simulink model "rmturretmodelrelease"  (R2025b)
settings: Solver=FixedStepAuto  StartTime=0.0  StopTime=tf  FixedStep=minstep  MaxStep=maxstep  MinStep=minstep  RelTol=tol  AbsTol=tol
values from neighbouring files (symbols this model uses):
  adecel = .4 * voltmax * kt * gearrat/(J * ra)    (= 19.7149704598)    [rmturretrelease.m]
  ascale = .9    (= 0.9)    [rmturretrelease.m]
  c = 5.526    [rmturretrelease.m]
  damp = .4    (= 0.4)    [rmturretrelease.m]
  dfreq = 3.7    [rmturretrelease.m]
  gearrat = 1    [rmturretrelease.m]
  intthresh = voltmax*.65    (= 15.6)    [rmturretrelease.m]
  ivmax = .8 / kiv    (= 0.016)    [rmturretrelease.m]
  J = 0.04145    [rmturretrelease.m]
  ka = J/(kt*gearrat)    (= 0.0559379217274)    [rmturretrelease.m]
  kb = .763 * g2    (= 0.763)    [rmturretrelease.m]
  kiv = 50    [rmturretrelease.m]
  kp = 23    [rmturretrelease.m]
  kpv = .01    (= 0.01)    [rmturretrelease.m]
  ks = uk /(kt*gearrat)    (= 1)    [rmturretrelease.m]
  kt = .741 * g2    (= 0.741)    [rmturretrelease.m]
  kv = kb*gearrat    (= 0.763)    [rmturretrelease.m]
  kvis = c/(kt*gearrat)    (= 7.45748987854)    [rmturretrelease.m]
  la = .00578 * 2    (= 0.01156)    [rmturretrelease.m]
  lat = .004    (= 0.004)    [rmturretrelease.m]
  namp = 0.0000000001    (= 1e-10)    [rmturretrelease.m]
  ra = 8.705    [rmturretrelease.m]
  squiggle = 0    [rmturretrelease.m]
  squigglefreq = 3    [rmturretrelease.m]
  testvel = 0    [rmturretrelease.m]
  theta0 = deg2rad(0)    [rmturretrelease.m]
  thetadotbreak = 6    [rmturretrelease.m]
  thetadotic = 0    [rmturretrelease.m]
  thetadotinput = 0    [rmturretrelease.m]
  thetatarget = deg2rad(170)    [rmturretrelease.m]
  Tpc = 1/500    (= 0.002)    [rmturretrelease.m]
  uk = .741    (= 0.741)    [rmturretrelease.m]
  vdt = 0    [rmturretrelease.m]
  veltar = 10    [rmturretrelease.m]
  vmax = voltmax /(kb * gearrat)    (= 31.4547837484)    [rmturretrelease.m]
  voltmax = 24    [rmturretrelease.m]
undefined symbols (not defined in the file or in its folder): DiscIntNeverNeededParam
libraries: simulink x6
settings Model: Creator=Localaccount  LastModifiedBy=Arihant
settings SolverCC: MaxConsecutiveZCs=10  ZeroCrossAlgorithm=Adaptive
settings DataIOCC: SaveOutput=off  SignalLogging=off  DSMLogging=off  SaveTime=off  ReturnWorkspaceOutputs=off
settings OptimizationCC: ZeroExternalMemoryAtStartup=off  ZeroInternalMemoryAtStartup=off
settings DebuggingCC: IgnoredZcDiagnostic=none
settings ModelReferenceCC: EnableRefExpFcnMdlSchedulingChecks=on
settings RTWCC: TargetLang=C++  GPUComputeCapability=3.5
settings GRTTargetCC: TargetLangStandard=C++11 (ISO)  CodeInterfacePackaging=C++ class  SubcomponentCodeInterfacePackaging=C++ class

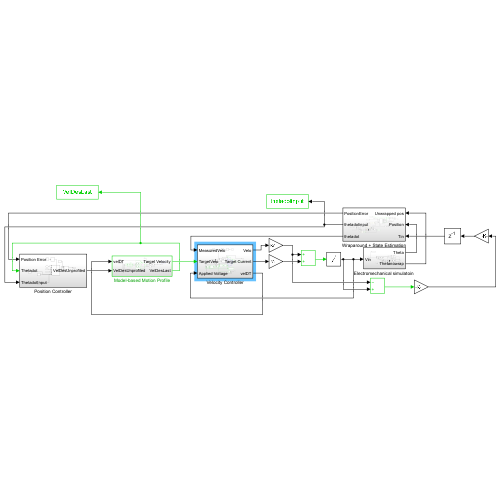
[thumbnail: Simulink's stored preview of the top-level diagram]
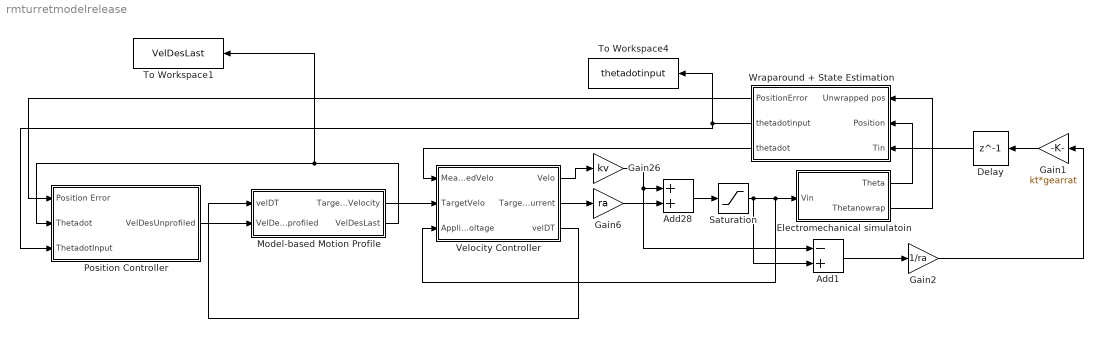
== system rmturretmodelrelease ==
  Add1 : Sum  Inputs=-+
  Add28 : Sum
  Delay : Delay  DelayLength=1  InitialCondition=0
  "Electromechanical simulatoin " : Subsystem
  Gain1 : Gain  Gain=kt*gearrat
  Gain2 : Gain  Gain=1/ra
  Gain26 : Gain  Gain=kv
  Gain6 : Gain  Gain=ra
  Model-based Motion Profile : Subsystem
  Position Controller : Subsystem
  Saturation : Saturate  UpperLimit=voltmax  LowerLimit=-voltmax
  To Workspace1 : ToWorkspace  VariableName=VelDesLast  SampleTime=-1
      settings: Save2DSignal=2-D array (concatenate along first dimension)
  To Workspace4 : ToWorkspace  VariableName=thetadotinput  SampleTime=-1
      settings: Save2DSignal=2-D array (concatenate along first dimension)
  Velocity Controller : Subsystem
  Wraparound + State Estimation : Subsystem
  wires:
  Gain26/1 -> Add1/1, Add28/1
  Gain6/1 -> Add28/2
  Add28/1 -> Saturation/1
  Saturation/1 -> Add1/2, Velocity Controller/3(Applied Voltage), "Electromechanical simulatoin "/1(Vin)
  Velocity Controller/3(velDT) -> Model-based Motion Profile/1(velDT)
  Wraparound + State Estimation/1(PositionError) -> Position Controller/1(Position Error)
  Model-based Motion Profile/1(Target Velocity) -> Velocity Controller/2(TargetVelo)
  Velocity Controller/1(Velo) -> Gain26/1
  Velocity Controller/2(Target Current) -> Gain6/1
  "Electromechanical simulatoin "/1(Theta) -> Wraparound + State Estimation/2(Position)
  "Electromechanical simulatoin "/2(Thetanowrap) -> Wraparound + State Estimation/1(Unwrapped pos)
  Position Controller/1(VelDesUnprofiled) -> Model-based Motion Profile/2(VelDesUnprofiled)
  Wraparound + State Estimation/2(thetadotinput) -> Position Controller/3(ThetadotInput), To Workspace4/1
  Model-based Motion Profile/2(VelDesLast) -> Position Controller/2(Thetadot), To Workspace1/1
  Wraparound + State Estimation/3(thetadot) -> Velocity Controller/1(MeasuredVelo)
  Gain1/1 -> Delay/1
  Gain2/1 -> Gain1/1
  Add1/1 -> Gain2/1
  Delay/1 -> Wraparound + State Estimation/3(Tin)

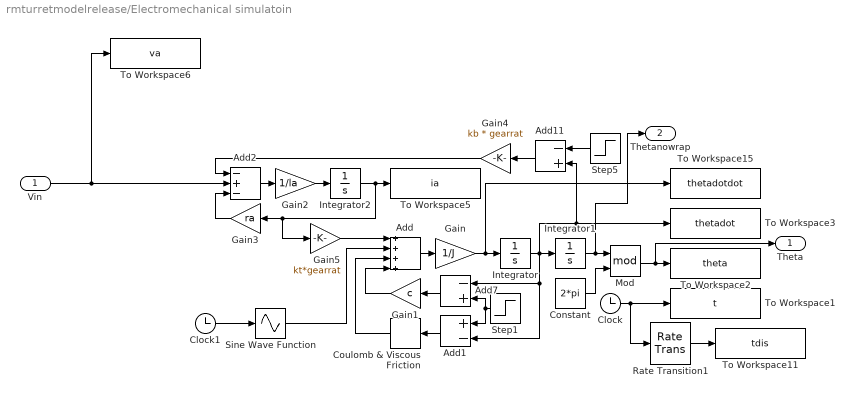
== system rmturretmodelrelease/Electromechanical simulatoin  ==
  Vin : Inport
  Add : Sum  Inputs=++++
  Add1 : Sum  Inputs=+-
  Add11 : Sum  Inputs=-+
  Add2 : Sum  Inputs=-+-
  Add7 : Sum  Inputs=-+
  Clock : Clock
  Clock1 : Clock
  Constant : Constant  Value=2*pi
  Coulomb & Viscous Friction : simulink/Discontinuities/Coulomb & Viscous Friction  offset=uk  gain=0
  Gain : Gain  Gain=1/J
  Gain1 : Gain  Gain=c
  Gain2 : Gain  Gain=1/la
  Gain3 : Gain  Gain=ra
  Gain4 : Gain  Gain=kb * gearrat
  Gain5 : Gain  Gain=kt*gearrat
  Integrator : Integrator  InitialCondition=thetadotic
  Integrator1 : Integrator  InitialCondition=theta0
  Integrator2 : Integrator
  Mod : Math  Operator=mod
  Rate Transition1 : RateTransition  OutPortSampleTime=Tpc
  Sine Wave Function : Sin  TimeSource=Use external signal  Amplitude=damp  Frequency=dfreq  SampleTime=0
  Step1 : Step  Time=0  After=vdt  SampleTime=0
  Step5 : Step  Time=0  After=vdt  SampleTime=0
  To Workspace1 : ToWorkspace  VariableName=t  SampleTime=-1
      settings: Save2DSignal=2-D array (concatenate along first dimension)
  To Workspace11 : ToWorkspace  VariableName=tdis  SampleTime=-1
      settings: Save2DSignal=2-D array (concatenate along first dimension)
  To Workspace15 : ToWorkspace  VariableName=thetadotdot  SampleTime=-1
      settings: Save2DSignal=2-D array (concatenate along first dimension)
  To Workspace2 : ToWorkspace  VariableName=theta  SampleTime=-1
      settings: Save2DSignal=2-D array (concatenate along first dimension)
  To Workspace3 : ToWorkspace  VariableName=thetadot  SampleTime=-1
      settings: Save2DSignal=2-D array (concatenate along first dimension)
  To Workspace5 : ToWorkspace  VariableName=ia  SampleTime=-1
      settings: Save2DSignal=2-D array (concatenate along first dimension)
  To Workspace6 : ToWorkspace  VariableName=va  SampleTime=-1
      settings: Save2DSignal=2-D array (concatenate along first dimension)
  Theta : Outport
  Thetanowrap : Outport  Port=2
  wires:
  Rate Transition1/1 -> To Workspace11/1
  Gain/1 -> To Workspace15/1, Integrator/1
  Constant/1 -> Mod/2
  Step1/1 -> Add1/1, Add7/2
  Add7/1 -> Gain1/1
  Gain4/1 -> Add2/1
  Integrator1/1 -> Thetanowrap/1, Mod/1
  Gain3/1 -> Add2/3
  Integrator/1 -> Integrator1/1, Add1/2, Add7/1, To Workspace3/1, Add11/2
  Add11/1 -> Gain4/1
  Add1/1 -> Coulomb & Viscous Friction/1
  Gain1/1 -> Add/4
  Sine Wave Function/1 -> Add/2
  Coulomb & Viscous Friction/1 -> Add/3
  Step5/1 -> Add11/1
  Integrator2/1 -> To Workspace5/1, Gain5/1, Gain3/1
  Mod/1 -> Theta/1, To Workspace2/1
  Gain5/1 -> Add/1
  Clock/1 -> To Workspace1/1, Rate Transition1/1
  Add2/1 -> Gain2/1
  Add/1 -> Gain/1
  Gain2/1 -> Integrator2/1
  Clock1/1 -> Sine Wave Function/1
  Vin/1 -> To Workspace6/1, Add2/2

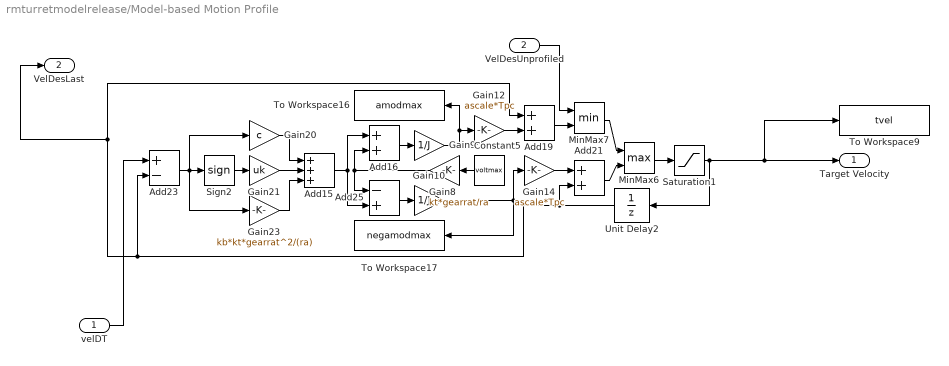
== system rmturretmodelrelease/Model-based Motion Profile ==
  velDT : Inport
  VelDesUnprofiled : Inport  Port=2
  Add15 : Sum  Inputs=+++
  Add16 : Sum
  Add19 : Sum
  Add21 : Sum
  Add23 : Sum  Inputs=+-
  Add25 : Sum  Inputs=-+
  Constant5 : Constant  Value=voltmax
  Gain10 : Gain  Gain=1/J
  Gain12 : Gain  Gain=ascale*Tpc
  Gain14 : Gain  Gain=ascale*Tpc
  Gain20 : Gain  Gain=c
  Gain21 : Gain  Gain=uk
  Gain23 : Gain  Gain=kb*kt*gearrat^2/(ra)
  Gain8 : Gain  Gain=kt*gearrat/ra
  Gain9 : Gain  Gain=1/J
  MinMax6 : MinMax  Function=max  Inputs=2
  MinMax7 : MinMax  Inputs=2
  Saturation1 : Saturate  UpperLimit=vmax  LowerLimit=-vmax
  Sign2 : Signum
  To Workspace16 : ToWorkspace  VariableName=amodmax  SampleTime=-1
      settings: Save2DSignal=2-D array (concatenate along first dimension)
  To Workspace17 : ToWorkspace  VariableName=negamodmax  SampleTime=-1
      settings: Save2DSignal=2-D array (concatenate along first dimension)
  To Workspace9 : ToWorkspace  VariableName=tvel  SampleTime=-1
      settings: Save2DSignal=2-D array (concatenate along first dimension)
  Unit Delay2 : UnitDelay  InitialCondition=thetadotic  SampleTime=Tpc  HasFrameUpgradeWarning=on
  Target Velocity : Outport
  VelDesLast : Outport  Port=2
  wires:
  Add21/1 -> MinMax6/2
  Saturation1/1 -> To Workspace9/1, Target Velocity/1, Unit Delay2/1
  Gain9/1 -> To Workspace16/1, Gain12/1
  Unit Delay2/1 -> Add21/2, Add23/2, VelDesLast/1, Add19/1
  Add15/1 -> Add16/1, Add25/2
  Gain14/1 -> Add21/1
  Gain23/1 -> Add15/3
  Constant5/1 -> Gain8/1
  Add19/1 -> MinMax7/2
  MinMax6/1 -> Saturation1/1
  Gain20/1 -> Add15/1
  Add23/1 -> Gain23/1, Gain20/1, Sign2/1
  Sign2/1 -> Gain21/1
  Gain10/1 -> Gain14/1, To Workspace17/1
  Add25/1 -> Gain10/1
  MinMax7/1 -> MinMax6/1
  Gain12/1 -> Add19/2
  Add16/1 -> Gain9/1
  Gain21/1 -> Add15/2
  Gain8/1 -> Add25/1, Add16/2
  VelDesUnprofiled/1 -> MinMax7/1
  velDT/1 -> Add23/1

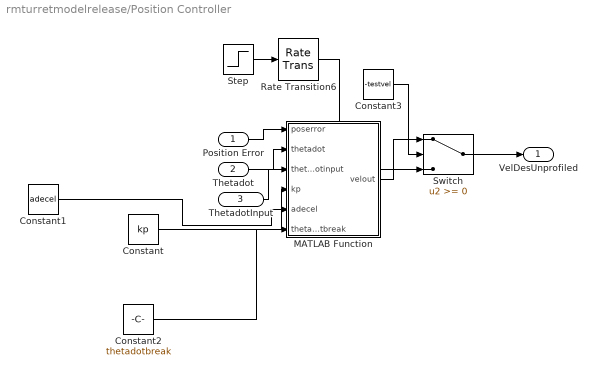
== system rmturretmodelrelease/Position Controller ==
  Position Error : Inport
  Thetadot : Inport  Port=2
  ThetadotInput : Inport  Port=3
  Constant : Constant  Value=kp
  Constant1 : Constant  Value=adecel
  Constant2 : Constant  Value=thetadotbreak
  Constant3 : Constant  Value=-testvel
  MATLAB Function : MATLAB Function  TreatAsAtomicUnit=on
  Rate Transition6 : RateTransition  OutPortSampleTime=Tpc
  Step : Step  Time=.05  After=veltar  SampleTime=0
  Switch : Switch  SaturateOnIntegerOverflow=off  InputSameDT=off
  VelDesUnprofiled : Outport
  wires:
  Position Error/1 -> MATLAB Function/1(poserror)
  Thetadot/1 -> MATLAB Function/2(thetadot)
  ThetadotInput/1 -> MATLAB Function/3(thetadotinput)
  Constant/1 -> MATLAB Function/4(kp)
  Constant1/1 -> MATLAB Function/5(adecel)
  Constant2/1 -> MATLAB Function/6(thetadotbreak)
  MATLAB Function/1(velout) -> Switch/1
  Switch/1 -> VelDesUnprofiled/1
  Constant3/1 -> Switch/2
  Step/1 -> Rate Transition6/1
  Rate Transition6/1 -> Switch/3

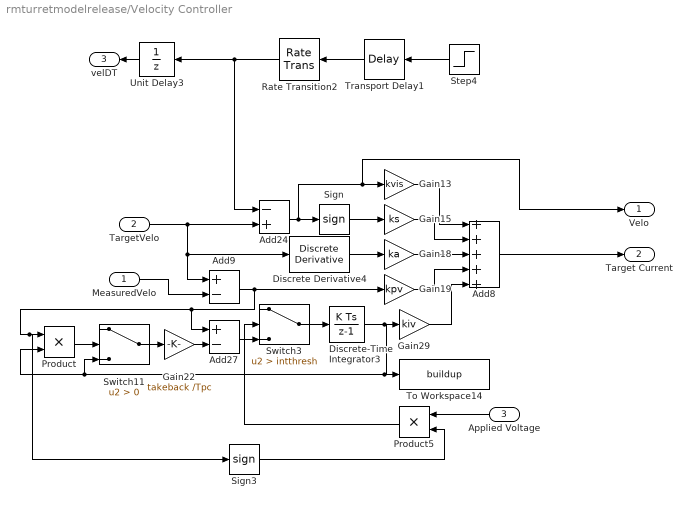
== system rmturretmodelrelease/Velocity Controller ==
  MeasuredVelo : Inport
  TargetVelo : Inport  Port=2
  Applied Voltage : Inport  Port=3
  Add24 : Sum  Inputs=-+
  Add27 : Sum  Inputs=+-
  Add8 : Sum  Inputs=+++++
  Add9 : Sum  Inputs=+-
  Discrete Derivative4 : simulink/Discrete/Discrete Derivative  gainval=1.0  ICPrevScaledInput=0.0  OutMin=[]  OutMax=[]  OutDataType=fixdt(1, 16)  OutScaling=2^-10  DoSatur=off
  Discrete-Time Integrator3 : DiscreteIntegrator  SampleTime=-1  LimitOutput=on  UpperSaturationLimit=ivmax  LowerSaturationLimit=-ivmax  ICPrevOutput=DiscIntNeverNeededParam  ICPrevScaledInput=DiscIntNeverNeededParam
  Gain13 : Gain  Gain=kvis
  Gain15 : Gain  Gain=ks
  Gain18 : Gain  Gain=ka
  Gain19 : Gain  Gain=kpv
  Gain22 : Gain  Gain=takeback /Tpc
  Gain29 : Gain  Gain=kiv
  Product : Product
  Product5 : Product
  Rate Transition2 : RateTransition  OutPortSampleTime=Tpc
  Sign : Signum
  Sign3 : Signum
  Step4 : Step  Time=0  After=vdt  SampleTime=0
  Switch11 : Switch  Criteria=u2 > Threshold  SaturateOnIntegerOverflow=off  InputSameDT=off
  Switch3 : Switch  Criteria=u2 > Threshold  Threshold=intthresh  SaturateOnIntegerOverflow=off  InputSameDT=off
  To Workspace14 : ToWorkspace  VariableName=buildup  SampleTime=-1
      settings: Save2DSignal=2-D array (concatenate along first dimension)
  Transport Delay1 : TransportDelay  DelayTime=lat
  Unit Delay3 : UnitDelay  SampleTime=Tpc  HasFrameUpgradeWarning=on
  Velo : Outport
  Target Current : Outport  Port=2
  velDT : Outport  Port=3
  wires:
  Applied Voltage/1 -> Product5/1
  Sign/1 -> Gain15/1
  Step4/1 -> Transport Delay1/1
  Transport Delay1/1 -> Rate Transition2/1
  Add24/1 -> Sign/1, Velo/1, Gain13/1
  Discrete-Time Integrator3/1 -> Product/2, Switch11/3, To Workspace14/1, Gain29/1
  Add9/1 -> Add27/1, Sign3/1, Product/1, Gain19/1
  Discrete Derivative4/1 -> Gain18/1
  Sign3/1 -> Product5/2
  TargetVelo/1 -> Add9/1, Discrete Derivative4/1, Add24/2
  Product5/1 -> Switch3/2
  Product/1 -> Switch11/2
  Add27/1 -> Switch3/3
  Gain13/1 -> Add8/1
  Gain18/1 -> Add8/3
  Gain15/1 -> Add8/2
  Switch11/1 -> Gain22/1
  Switch3/1 -> Discrete-Time Integrator3/1
  Rate Transition2/1 -> Add24/1, Unit Delay3/1
  Gain29/1 -> Add8/5
  Gain22/1 -> Add27/2
  Gain19/1 -> Add8/4
  MeasuredVelo/1 -> Add9/2
  Add8/1 -> Target Current/1
  Unit Delay3/1 -> velDT/1

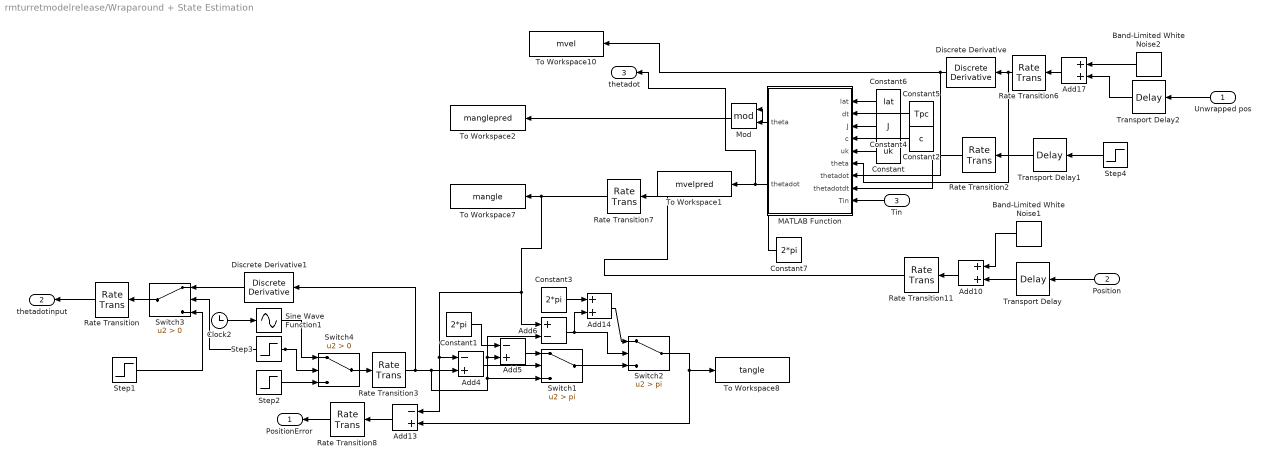
== system rmturretmodelrelease/Wraparound + State Estimation ==
  Unwrapped pos : Inport
  Position : Inport  Port=2
  Tin : Inport  Port=3
  Add10 : Sum
  Add13 : Sum  Inputs=-+
  Add14 : Sum
  Add17 : Sum
  Add4 : Sum  Inputs=-+
  Add5 : Sum  Inputs=-+
  Add6 : Sum  Inputs=+-
  Band-Limited White Noise1 : simulink/Sources/Band-Limited White Noise  Cov=[namp]  Ts=0.01  seed=[23341]
  Band-Limited White Noise2 : simulink/Sources/Band-Limited White Noise  Cov=[namp]  Ts=0.01  seed=[23341]
  Clock2 : Clock
  Constant : Constant  Value=uk
  Constant1 : Constant  Value=2*pi
  Constant2 : Constant  Value=c
  Constant3 : Constant  Value=2*pi
  Constant4 : Constant  Value=J
  Constant5 : Constant  Value=Tpc
  Constant6 : Constant  Value=lat
  Constant7 : Constant  Value=2*pi
  Discrete Derivative : simulink/Discrete/Discrete Derivative  gainval=1.0  ICPrevScaledInput=0.0  OutMin=[]  OutMax=[]  OutDataType=fixdt(1, 16)  OutScaling=2^-10  DoSatur=off
  Discrete Derivative1 : simulink/Discrete/Discrete Derivative  gainval=1.0  ICPrevScaledInput=0.0  OutMin=[]  OutMax=[]  OutDataType=fixdt(1, 16)  OutScaling=2^-10  DoSatur=off
  MATLAB Function : MATLAB Function  TreatAsAtomicUnit=on
  Mod : Math  Operator=mod
  Rate Transition{,2..3,6..8,11} (7 alike) : RateTransition  OutPortSampleTime=Tpc
  Sine Wave Function1 : Sin  TimeSource=Use external signal  Amplitude=thetatarget  Bias=pi  Frequency=squigglefreq  SampleTime=0
  Step1 : Step  Time=lat  After=thetadotinput  SampleTime=0
  Step2 : Step  Time=lat  After=thetatarget  SampleTime=0
  Step3 : Step  Time=lat  After=squiggle  SampleTime=0
  Step4 : Step  Time=0  After=vdt  SampleTime=0
  Switch1 : Switch  Criteria=u2 > Threshold  Threshold=pi  SaturateOnIntegerOverflow=off  InputSameDT=off
  Switch2 : Switch  Criteria=u2 > Threshold  Threshold=pi  SaturateOnIntegerOverflow=off  InputSameDT=off
  Switch3 : Switch  Criteria=u2 > Threshold  SaturateOnIntegerOverflow=off  InputSameDT=off
  Switch4 : Switch  Criteria=u2 > Threshold  SaturateOnIntegerOverflow=off  InputSameDT=off
  To Workspace1 : ToWorkspace  VariableName=mvelpred  SampleTime=-1
      settings: Save2DSignal=2-D array (concatenate along first dimension)
  To Workspace10 : ToWorkspace  VariableName=mvel  SampleTime=-1
      settings: Save2DSignal=2-D array (concatenate along first dimension)
  To Workspace2 : ToWorkspace  VariableName=manglepred  SampleTime=-1
      settings: Save2DSignal=2-D array (concatenate along first dimension)
  To Workspace7 : ToWorkspace  VariableName=mangle  SampleTime=-1
      settings: Save2DSignal=2-D array (concatenate along first dimension)
  To Workspace8 : ToWorkspace  VariableName=tangle  SampleTime=-1
      settings: Save2DSignal=2-D array (concatenate along first dimension)
  Transport Delay : TransportDelay  DelayTime=lat
  Transport Delay1 : TransportDelay  DelayTime=lat
  Transport Delay2 : TransportDelay  DelayTime=lat
  PositionError : Outport
  thetadotinput : Outport  Port=2
  thetadot : Outport  Port=3
  wires:
  Transport Delay/1 -> Add10/2
  Rate Transition3/1 -> Discrete Derivative1/1, Add5/2, Add6/2, Switch1/3, Add4/2
  Add4/1 -> Switch1/2
  Rate Transition11/1 -> Rate Transition7/1
  Switch4/1 -> Rate Transition3/1
  Constant1/1 -> Add5/1
  Sine Wave Function1/1 -> Switch4/1
  Step3/1 -> Switch4/2, Switch3/2
  Switch1/1 -> Switch2/3
  Constant3/1 -> Add14/1
  Transport Delay2/1 -> Add17/2
  Add5/1 -> Switch1/1
  Band-Limited White Noise2/1 -> Add17/1
  Add13/1 -> Rate Transition8/1
  Switch2/1 -> Add13/2, To Workspace8/1
  Band-Limited White Noise1/1 -> Add10/1
  Discrete Derivative/1 -> To Workspace10/1, MATLAB Function/7("thetadot ")
  Add14/1 -> Switch2/1
  Add6/1 -> Switch2/2, Add14/2
  Clock2/1 -> Sine Wave Function1/1
  Add10/1 -> Rate Transition11/1
  Unwrapped pos/1 -> Transport Delay2/1
  Rate Transition7/1 -> Add6/1, Add13/1, Add4/1, To Workspace7/1
  Add17/1 -> Rate Transition6/1
  Rate Transition6/1 -> MATLAB Function/6("theta "), Discrete Derivative/1
  Position/1 -> Transport Delay/1
  Rate Transition8/1 -> PositionError/1
  Discrete Derivative1/1 -> Switch3/1
  Switch3/1 -> Rate Transition/1
  Step2/1 -> Switch4/3
  Step1/1 -> Switch3/3
  Rate Transition/1 -> thetadotinput/1
  Transport Delay1/1 -> Rate Transition2/1
  Step4/1 -> Transport Delay1/1
  Rate Transition2/1 -> MATLAB Function/8(thetadotdt)
  Tin/1 -> MATLAB Function/9(Tin)
  Constant/1 -> MATLAB Function/5(uk)
  Constant2/1 -> MATLAB Function/4(c)
  Constant4/1 -> MATLAB Function/3(J)
  Constant5/1 -> MATLAB Function/2(dt)
  Constant6/1 -> MATLAB Function/1(lat)
  MATLAB Function/1(theta) -> Mod/1
  Mod/1 -> To Workspace2/1
  Constant7/1 -> Mod/2
  MATLAB Function/2(thetadot) -> thetadot/1, To Workspace1/1

== matlab function rmturretmodelrelease/Wraparound + State Estimation/MATLAB Function ==
  data: lat input; theta output; dt input; J input; c input; uk input; theta input; thetadot input; thetadotdt input; Tin input; thetadot output
%TODO: ADD FILTERING THEORY TO MAKE ROBUST

function [theta, thetadot] = fcn(lat, dt, J, c, uk, theta, thetadot, thetadotdt, Tin)

persistent Tqueue

%Queue singletons
if isempty(Tqueue)
    Tqueue = [0 0 0 0];
end

Tqueue = [Tqueue(2:end), Tin];

for i = 1:lat/dt
   thetadot = thetadot + (Tqueue(i) - c*(thetadot - thetadotdt) - uk*sign(thetadot - thetadotdt))*dt/J;
   theta = theta + thetadot*dt;
end

== matlab function rmturretmodelrelease/Position Controller/MATLAB Function ==
  data: poserror input; velout output; thetadot input; thetadotinput input; kp input; adecel input; thetadotbreak input
function velout  = fcn(poserror, thetadot, thetadotinput, kp, adecel, thetadotbreak)

o = 0;
o2 = 0;
if abs(thetadotinput) > thetadotbreak
 % o = (thetadotinput - thetadotbreak)/kp + (thetadotbreak^2 - thetadotinput^2) / (2*adecel);
 % o2 = (thetadotinput + thetadotbreak)/kp + (thetadotinput^2 - thetadotbreak^2) / (2*adecel);
end

v1 = 0;
v2 = 0;
v3 = 0;
v4 = 0;

if thetadotinput^2 - 2*adecel*(-poserror - o) >= 0
    v1 = sqrt(thetadotinput^2 - 2*adecel*(-poserror - o)); %Positive left
    v2 = -sqrt(thetadotinput^2 - 2*adecel*(-poserror - o)); %Negative left
end
if thetadotinput^2 - 2*adecel*(poserror + o2) >= 0
    v3 = sqrt(thetadotinput^2 - 2*adecel*(poserror + o2)); %Positive right
    v4 = -sqrt(thetadotinput^2 - 2*adecel*(poserror + o2)); %Negative right
end
    if poserror < thetadotbreak/kp
        v = kp*poserror + thetadotinput;
    elseif (v3 ~= 0 && poserror > 0 && thetadot <= 0)
        v = v3;
    elseif (v2 ~= 0 && poserror < 0 && thetadot >= 0)
        v = v2;
    elseif poserror > 0
        v = v1;
    else
        v = v4;
    end
    

velout = v;
